simulink model "dandianji"  (R2014b)
settings: Solver=ode45  StartTime=0.0  StopTime=10.0  RelTol=1e-3
undefined symbols (not defined in the file): sigbuilder_block
libraries: simulink x33, fuzblock x16
(part 1 of 2)
settings Model: Creator=Administrator  LastModifiedBy=Administrator

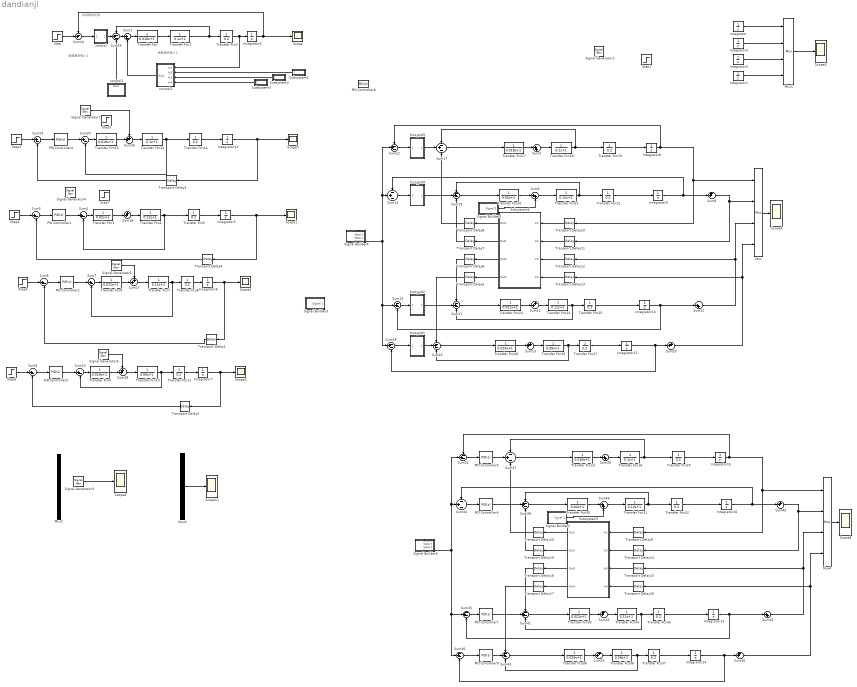
== system dandianji ==
  note: 偏差耦合输入2
  note: 系统原有反馈
  note: 偏差耦合输入1
  Integrator{,1..16} (17 alike) : Integrator
  Mux{,1..4} (5 alike) : Mux
  PID Controller1 : simulink/Continuous/PID Controller  Controller=PID  TimeDomain=Continuous-time  SampleTime=-1  IntegratorMethod=Forward Euler  FilterMethod=Forward Euler  Form=Parallel  P=4.34348893595362  I=0.409606906541511  D=0.190106280421876  N=113.521570556965  InitialConditionSource=internal  InitialConditionForIntegrator=0  InitialConditionForFilter=0  ExternalReset=none  LimitOutput=off  UpperSaturationLimit=inf  LowerSaturationLimit=-inf  LinearizeAsGain=on  AntiWindupMode=none  Kb=1  TrackingMode=off  Kt=1  PParamMin=[]  PParamMax=[]  IParamMin=[]  IParamMax=[]  DParamMin=[]  DParamMax=[]  NParamMin=[]  NParamMax=[]  KbParamMin=[]  KbParamMax=[]  KtParamMin=[]  KtParamMax=[]  POutMin=[]  POutMax=[]  IOutMin=[]  IOutMax=[]  DOutMin=[]  DOutMax=[]  NOutMin=[]  NOutMax=[]  KbOutMin=[]  KbOutMax=[]  KtOutMin=[]  KtOutMax=[]  IntegratorOutMin=[]  IntegratorOutMax=[]  FilterOutMin=[]  FilterOutMax=[]  SumOutMin=[]  SumOutMax=[]  SumI1OutMin=[]  SumI1OutMax=[]  SumI2OutMin=[]  SumI2OutMax=[]  SumI3OutMin=[]  SumI3OutMax=[]  SumDOutMin=[]  SumDOutMax=[]  SaturationOutMin=[]  SaturationOutMax=[]  IntegratorContinuousStateAttributes=''  IntegratorStateMustResolveToSignalObject=off  IntegratorRTWStateStorageClass=Auto  FilterContinuousStateAttributes=''  FilterStateMustResolveToSignalObject=off  FilterRTWStateStorageClass=Auto  DifferentiatorICPrevScaledInput=0  DifferentiatorOutMin=[]  DifferentiatorOutMax=[]  UseFilter=on
  PID Controller2 : simulink/Continuous/PID Controller  Controller=PID  TimeDomain=Continuous-time  SampleTime=-1  IntegratorMethod=Forward Euler  FilterMethod=Forward Euler  Form=Parallel  P=4.3714761921553  I=0.418612157121434  D=0.176716531069936  N=115.244644738995  InitialConditionSource=internal  InitialConditionForIntegrator=0  InitialConditionForFilter=0  ExternalReset=none  LimitOutput=off  UpperSaturationLimit=inf  LowerSaturationLimit=-inf  LinearizeAsGain=on  AntiWindupMode=none  Kb=1  TrackingMode=off  Kt=1  PParamMin=[]  PParamMax=[]  IParamMin=[]  IParamMax=[]  DParamMin=[]  DParamMax=[]  NParamMin=[]  NParamMax=[]  KbParamMin=[]  KbParamMax=[]  KtParamMin=[]  KtParamMax=[]  POutMin=[]  POutMax=[]  IOutMin=[]  IOutMax=[]  DOutMin=[]  DOutMax=[]  NOutMin=[]  NOutMax=[]  KbOutMin=[]  KbOutMax=[]  KtOutMin=[]  KtOutMax=[]  IntegratorOutMin=[]  IntegratorOutMax=[]  FilterOutMin=[]  FilterOutMax=[]  SumOutMin=[]  SumOutMax=[]  SumI1OutMin=[]  SumI1OutMax=[]  SumI2OutMin=[]  SumI2OutMax=[]  SumI3OutMin=[]  SumI3OutMax=[]  SumDOutMin=[]  SumDOutMax=[]  SaturationOutMin=[]  SaturationOutMax=[]  IntegratorContinuousStateAttributes=''  IntegratorStateMustResolveToSignalObject=off  IntegratorRTWStateStorageClass=Auto  FilterContinuousStateAttributes=''  FilterStateMustResolveToSignalObject=off  FilterRTWStateStorageClass=Auto  DifferentiatorICPrevScaledInput=0  DifferentiatorOutMin=[]  DifferentiatorOutMax=[]  UseFilter=on
  PID Controller3 : simulink/Continuous/PID Controller  Controller=PID  TimeDomain=Continuous-time  SampleTime=-1  IntegratorMethod=Forward Euler  FilterMethod=Forward Euler  Form=Parallel  P=4.54060551459518  I=0.450019772467081  D=0.137661903224342  N=119.172045893014  InitialConditionSource=internal  InitialConditionForIntegrator=0  InitialConditionForFilter=0  ExternalReset=none  LimitOutput=off  UpperSaturationLimit=inf  LowerSaturationLimit=-inf  LinearizeAsGain=on  AntiWindupMode=none  Kb=1  TrackingMode=off  Kt=1  PParamMin=[]  PParamMax=[]  IParamMin=[]  IParamMax=[]  DParamMin=[]  DParamMax=[]  NParamMin=[]  NParamMax=[]  KbParamMin=[]  KbParamMax=[]  KtParamMin=[]  KtParamMax=[]  POutMin=[]  POutMax=[]  IOutMin=[]  IOutMax=[]  DOutMin=[]  DOutMax=[]  NOutMin=[]  NOutMax=[]  KbOutMin=[]  KbOutMax=[]  KtOutMin=[]  KtOutMax=[]  IntegratorOutMin=[]  IntegratorOutMax=[]  FilterOutMin=[]  FilterOutMax=[]  SumOutMin=[]  SumOutMax=[]  SumI1OutMin=[]  SumI1OutMax=[]  SumI2OutMin=[]  SumI2OutMax=[]  SumI3OutMin=[]  SumI3OutMax=[]  SumDOutMin=[]  SumDOutMax=[]  SaturationOutMin=[]  SaturationOutMax=[]  IntegratorContinuousStateAttributes=''  IntegratorStateMustResolveToSignalObject=off  IntegratorRTWStateStorageClass=Auto  FilterContinuousStateAttributes=''  FilterStateMustResolveToSignalObject=off  FilterRTWStateStorageClass=Auto  DifferentiatorICPrevScaledInput=0  DifferentiatorOutMin=[]  DifferentiatorOutMax=[]  UseFilter=on
  PID Controller4 : simulink/Continuous/PID Controller  Controller=PID  TimeDomain=Continuous-time  SampleTime=-1  IntegratorMethod=Forward Euler  FilterMethod=Forward Euler  Form=Parallel  P=4.45385591758043  I=0.428539114293849  D=0.147050814476134  N=115.714109449814  InitialConditionSource=internal  InitialConditionForIntegrator=0  InitialConditionForFilter=0  ExternalReset=none  LimitOutput=off  UpperSaturationLimit=inf  LowerSaturationLimit=-inf  LinearizeAsGain=on  AntiWindupMode=none  Kb=1  TrackingMode=off  Kt=1  PParamMin=[]  PParamMax=[]  IParamMin=[]  IParamMax=[]  DParamMin=[]  DParamMax=[]  NParamMin=[]  NParamMax=[]  KbParamMin=[]  KbParamMax=[]  KtParamMin=[]  KtParamMax=[]  POutMin=[]  POutMax=[]  IOutMin=[]  IOutMax=[]  DOutMin=[]  DOutMax=[]  NOutMin=[]  NOutMax=[]  KbOutMin=[]  KbOutMax=[]  KtOutMin=[]  KtOutMax=[]  IntegratorOutMin=[]  IntegratorOutMax=[]  FilterOutMin=[]  FilterOutMax=[]  SumOutMin=[]  SumOutMax=[]  SumI1OutMin=[]  SumI1OutMax=[]  SumI2OutMin=[]  SumI2OutMax=[]  SumI3OutMin=[]  SumI3OutMax=[]  SumDOutMin=[]  SumDOutMax=[]  SaturationOutMin=[]  SaturationOutMax=[]  IntegratorContinuousStateAttributes=''  IntegratorStateMustResolveToSignalObject=off  IntegratorRTWStateStorageClass=Auto  FilterContinuousStateAttributes=''  FilterStateMustResolveToSignalObject=off  FilterRTWStateStorageClass=Auto  DifferentiatorICPrevScaledInput=0  DifferentiatorOutMin=[]  DifferentiatorOutMax=[]  UseFilter=on
  PID Controller5 : simulink/Continuous/PID Controller  Controller=PID  TimeDomain=Continuous-time  SampleTime=-1  IntegratorMethod=Forward Euler  FilterMethod=Forward Euler  Form=Parallel  P=4.45385591758043  I=0.428539114293849  D=0.147050814476134  N=115.714109449814  InitialConditionSource=internal  InitialConditionForIntegrator=0  InitialConditionForFilter=0  ExternalReset=none  LimitOutput=off  UpperSaturationLimit=inf  LowerSaturationLimit=-inf  LinearizeAsGain=on  AntiWindupMode=none  Kb=1  TrackingMode=off  Kt=1  PParamMin=[]  PParamMax=[]  IParamMin=[]  IParamMax=[]  DParamMin=[]  DParamMax=[]  NParamMin=[]  NParamMax=[]  KbParamMin=[]  KbParamMax=[]  KtParamMin=[]  KtParamMax=[]  POutMin=[]  POutMax=[]  IOutMin=[]  IOutMax=[]  DOutMin=[]  DOutMax=[]  NOutMin=[]  NOutMax=[]  KbOutMin=[]  KbOutMax=[]  KtOutMin=[]  KtOutMax=[]  IntegratorOutMin=[]  IntegratorOutMax=[]  FilterOutMin=[]  FilterOutMax=[]  SumOutMin=[]  SumOutMax=[]  SumI1OutMin=[]  SumI1OutMax=[]  SumI2OutMin=[]  SumI2OutMax=[]  SumI3OutMin=[]  SumI3OutMax=[]  SumDOutMin=[]  SumDOutMax=[]  SaturationOutMin=[]  SaturationOutMax=[]  IntegratorContinuousStateAttributes=''  IntegratorStateMustResolveToSignalObject=off  IntegratorRTWStateStorageClass=Auto  FilterContinuousStateAttributes=''  FilterStateMustResolveToSignalObject=off  FilterRTWStateStorageClass=Auto  DifferentiatorICPrevScaledInput=0  DifferentiatorOutMin=[]  DifferentiatorOutMax=[]  UseFilter=on
  PID Controller6 : simulink/Continuous/PID Controller  Controller=PID  TimeDomain=Continuous-time  SampleTime=-1  IntegratorMethod=Forward Euler  FilterMethod=Forward Euler  Form=Parallel  P=4.34348893595362  I=0.409606906541511  D=0.190106280421876  N=113.521570556965  InitialConditionSource=internal  InitialConditionForIntegrator=0  InitialConditionForFilter=0  ExternalReset=none  LimitOutput=off  UpperSaturationLimit=inf  LowerSaturationLimit=-inf  LinearizeAsGain=on  AntiWindupMode=none  Kb=1  TrackingMode=off  Kt=1  PParamMin=[]  PParamMax=[]  IParamMin=[]  IParamMax=[]  DParamMin=[]  DParamMax=[]  NParamMin=[]  NParamMax=[]  KbParamMin=[]  KbParamMax=[]  KtParamMin=[]  KtParamMax=[]  POutMin=[]  POutMax=[]  IOutMin=[]  IOutMax=[]  DOutMin=[]  DOutMax=[]  NOutMin=[]  NOutMax=[]  KbOutMin=[]  KbOutMax=[]  KtOutMin=[]  KtOutMax=[]  IntegratorOutMin=[]  IntegratorOutMax=[]  FilterOutMin=[]  FilterOutMax=[]  SumOutMin=[]  SumOutMax=[]  SumI1OutMin=[]  SumI1OutMax=[]  SumI2OutMin=[]  SumI2OutMax=[]  SumI3OutMin=[]  SumI3OutMax=[]  SumDOutMin=[]  SumDOutMax=[]  SaturationOutMin=[]  SaturationOutMax=[]  IntegratorContinuousStateAttributes=''  IntegratorStateMustResolveToSignalObject=off  IntegratorRTWStateStorageClass=Auto  FilterContinuousStateAttributes=''  FilterStateMustResolveToSignalObject=off  FilterRTWStateStorageClass=Auto  DifferentiatorICPrevScaledInput=0  DifferentiatorOutMin=[]  DifferentiatorOutMax=[]  UseFilter=on
  PID Controller7 : simulink/Continuous/PID Controller  Controller=PID  TimeDomain=Continuous-time  SampleTime=-1  IntegratorMethod=Forward Euler  FilterMethod=Forward Euler  Form=Parallel  P=4.3714761921553  I=0.418612157121434  D=0.176716531069936  N=115.244644738995  InitialConditionSource=internal  InitialConditionForIntegrator=0  InitialConditionForFilter=0  ExternalReset=none  LimitOutput=off  UpperSaturationLimit=inf  LowerSaturationLimit=-inf  LinearizeAsGain=on  AntiWindupMode=none  Kb=1  TrackingMode=off  Kt=1  PParamMin=[]  PParamMax=[]  IParamMin=[]  IParamMax=[]  DParamMin=[]  DParamMax=[]  NParamMin=[]  NParamMax=[]  KbParamMin=[]  KbParamMax=[]  KtParamMin=[]  KtParamMax=[]  POutMin=[]  POutMax=[]  IOutMin=[]  IOutMax=[]  DOutMin=[]  DOutMax=[]  NOutMin=[]  NOutMax=[]  KbOutMin=[]  KbOutMax=[]  KtOutMin=[]  KtOutMax=[]  IntegratorOutMin=[]  IntegratorOutMax=[]  FilterOutMin=[]  FilterOutMax=[]  SumOutMin=[]  SumOutMax=[]  SumI1OutMin=[]  SumI1OutMax=[]  SumI2OutMin=[]  SumI2OutMax=[]  SumI3OutMin=[]  SumI3OutMax=[]  SumDOutMin=[]  SumDOutMax=[]  SaturationOutMin=[]  SaturationOutMax=[]  IntegratorContinuousStateAttributes=''  IntegratorStateMustResolveToSignalObject=off  IntegratorRTWStateStorageClass=Auto  FilterContinuousStateAttributes=''  FilterStateMustResolveToSignalObject=off  FilterRTWStateStorageClass=Auto  DifferentiatorICPrevScaledInput=0  DifferentiatorOutMin=[]  DifferentiatorOutMax=[]  UseFilter=on
  PID Controller8 : simulink/Continuous/PID Controller  Controller=PID  TimeDomain=Continuous-time  SampleTime=-1  IntegratorMethod=Forward Euler  FilterMethod=Forward Euler  Form=Parallel  P=12.9851074749726  I=3.96505413373294  D=0.756963167778154  N=4061.73491108422  InitialConditionSource=internal  InitialConditionForIntegrator=0  InitialConditionForFilter=0  ExternalReset=none  LimitOutput=off  UpperSaturationLimit=inf  LowerSaturationLimit=-inf  LinearizeAsGain=on  AntiWindupMode=none  Kb=1  TrackingMode=off  Kt=1  PParamMin=[]  PParamMax=[]  IParamMin=[]  IParamMax=[]  DParamMin=[]  DParamMax=[]  NParamMin=[]  NParamMax=[]  KbParamMin=[]  KbParamMax=[]  KtParamMin=[]  KtParamMax=[]  POutMin=[]  POutMax=[]  IOutMin=[]  IOutMax=[]  DOutMin=[]  DOutMax=[]  NOutMin=[]  NOutMax=[]  KbOutMin=[]  KbOutMax=[]  KtOutMin=[]  KtOutMax=[]  IntegratorOutMin=[]  IntegratorOutMax=[]  FilterOutMin=[]  FilterOutMax=[]  SumOutMin=[]  SumOutMax=[]  SumI1OutMin=[]  SumI1OutMax=[]  SumI2OutMin=[]  SumI2OutMax=[]  SumI3OutMin=[]  SumI3OutMax=[]  SumDOutMin=[]  SumDOutMax=[]  SaturationOutMin=[]  SaturationOutMax=[]  IntegratorContinuousStateAttributes=''  IntegratorStateMustResolveToSignalObject=off  IntegratorRTWStateStorageClass=Auto  FilterContinuousStateAttributes=''  FilterStateMustResolveToSignalObject=off  FilterRTWStateStorageClass=Auto  DifferentiatorICPrevScaledInput=0  DifferentiatorOutMin=[]  DifferentiatorOutMax=[]  UseFilter=on
  PID Controller9 : simulink/Continuous/PID Controller  Controller=PID  TimeDomain=Continuous-time  SampleTime=-1  IntegratorMethod=Forward Euler  FilterMethod=Forward Euler  Form=Parallel  P=4.54060551459518  I=0.450019772467081  D=0.137661903224342  N=119.172045893014  InitialConditionSource=internal  InitialConditionForIntegrator=0  InitialConditionForFilter=0  ExternalReset=none  LimitOutput=off  UpperSaturationLimit=inf  LowerSaturationLimit=-inf  LinearizeAsGain=on  AntiWindupMode=none  Kb=1  TrackingMode=off  Kt=1  PParamMin=[]  PParamMax=[]  IParamMin=[]  IParamMax=[]  DParamMin=[]  DParamMax=[]  NParamMin=[]  NParamMax=[]  KbParamMin=[]  KbParamMax=[]  KtParamMin=[]  KtParamMax=[]  POutMin=[]  POutMax=[]  IOutMin=[]  IOutMax=[]  DOutMin=[]  DOutMax=[]  NOutMin=[]  NOutMax=[]  KbOutMin=[]  KbOutMax=[]  KtOutMin=[]  KtOutMax=[]  IntegratorOutMin=[]  IntegratorOutMax=[]  FilterOutMin=[]  FilterOutMax=[]  SumOutMin=[]  SumOutMax=[]  SumI1OutMin=[]  SumI1OutMax=[]  SumI2OutMin=[]  SumI2OutMax=[]  SumI3OutMin=[]  SumI3OutMax=[]  SumDOutMin=[]  SumDOutMax=[]  SaturationOutMin=[]  SaturationOutMax=[]  IntegratorContinuousStateAttributes=''  IntegratorStateMustResolveToSignalObject=off  IntegratorRTWStateStorageClass=Auto  FilterContinuousStateAttributes=''  FilterStateMustResolveToSignalObject=off  FilterRTWStateStorageClass=Auto  DifferentiatorICPrevScaledInput=0  DifferentiatorOutMin=[]  DifferentiatorOutMax=[]  UseFilter=on
  Scope{,1..8,11} (10 alike) : Scope
      Scope settings: SaveName=dianji1
      Scope1 settings: SaveName=dianji2
      Scope11 settings: YMin=260  YMax=460  SaveName=wuraodongweizhi5
      Scope2 settings: SaveName=dianji3
      Scope3 settings: SaveName=dianji4
      Scope4 settings: YMin=4.94  YMax=5.02  SaveName=perfect
      Scope5 settings: YMin=260  YMax=460  SaveName=wuraodongweizhi
      Scope6 settings: YMin=-500  YMax=2000  SaveName=wuraodongweizhi1
      Scope7 settings: SaveName=dianji
      Scope8 settings: YMin=4.7  YMax=5.4  SaveName=perfect1
  Signal Generator{1,4..6} (4 alike) : SignalGenerator  WaveForm=random  Amplitude=10  Frequency=2
  Signal Generator2 : SignalGenerator  WaveForm=random  Frequency=2
  Signal Generator3 : SignalGenerator  WaveForm=random  Frequency=2
  Signal Builder1 : Subsystem  Tag=STV Subsys  LoadFcn=sigbuilder_block('load');  StartFcn=sigbuilder_block('start');  StopFcn=sigbuilder_block('stop');  ClipboardFcn=sigbuilder_block('clipboard');  mask(Sigbuilder block){}
      mask help: Simulink:masks:SigbuilderBlock_MD
      mask init:
      | if ~strcmp(get_param(bdroot(gcbh),'SimulationStatus'),'stopped') tuvar = sigbuilder_block('maskInit'); end
      settings: CopyFcn=sigbuilder_block('copy');  DeleteFcn=sigbuilder_block('delete');  ModelCloseFcn=sigbuilder_block('modelClose');  PreSaveFcn=sigbuilder_block('preSave');  PauseFcn=sigbuilder_block('pause');  ContinueFcn=sigbuilder_block('continue');  NameChangeFcn=sigbuilder_block('namechange');  OpenFcn=sigbuilder_block('open',[437.6 199.2 550.4 400 ]);  CloseFcn=sigbuilder_block('close');
      mask Display: plot(0, 0, 100, 100,[2, 2, 32, 32, 2], [68, 8, 8, 68, 68],[32, 2], [38, 38], [32, 19, 2],[53, 60, 44], [32, 17, 17, 2],[16, 16, 31, 31]);txt = getActiveGroup(gcbh);text(2, 100, txt,'verticalAlignment', 'top');
  Signal Builder2 : Subsystem  Tag=STV Subsys  LoadFcn=sigbuilder_block('load');  StartFcn=sigbuilder_block('start');  StopFcn=sigbuilder_block('stop');  ClipboardFcn=sigbuilder_block('clipboard');  mask(Sigbuilder block){}
      mask help: Simulink:masks:SigbuilderBlock_MD
      mask init:
      | if ~strcmp(get_param(bdroot(gcbh),'SimulationStatus'),'stopped') tuvar = sigbuilder_block('maskInit'); end
      settings: CopyFcn=sigbuilder_block('copy');  DeleteFcn=sigbuilder_block('delete');  ModelCloseFcn=sigbuilder_block('modelClose');  PreSaveFcn=sigbuilder_block('preSave');  PauseFcn=sigbuilder_block('pause');  ContinueFcn=sigbuilder_block('continue');  NameChangeFcn=sigbuilder_block('namechange');  OpenFcn=sigbuilder_block('open',[437.6 199.2 550.4 400 ]);  CloseFcn=sigbuilder_block('close');
      mask Display: plot(0, 0, 100, 100,[2, 2, 32, 32, 2], [68, 8, 8, 68, 68],[32, 2], [38, 38], [32, 19, 2],[53, 60, 44], [32, 17, 17, 2],[16, 16, 31, 31]);txt = getActiveGroup(gcbh);text(2, 100, txt,'verticalAlignment', 'top');
  Signal Builder3 : Subsystem  Tag=STV Subsys  LoadFcn=sigbuilder_block('load');  StartFcn=sigbuilder_block('start');  StopFcn=sigbuilder_block('stop');  ClipboardFcn=sigbuilder_block('clipboard');  mask(Sigbuilder block){}
      mask help: Simulink:masks:SigbuilderBlock_MD
      mask init:
      | if ~strcmp(get_param(bdroot(gcbh),'SimulationStatus'),'stopped') tuvar = sigbuilder_block('maskInit'); end
      settings: CopyFcn=sigbuilder_block('copy');  DeleteFcn=sigbuilder_block('delete');  ModelCloseFcn=sigbuilder_block('modelClose');  PreSaveFcn=sigbuilder_block('preSave');  PauseFcn=sigbuilder_block('pause');  ContinueFcn=sigbuilder_block('continue');  NameChangeFcn=sigbuilder_block('namechange');  OpenFcn=sigbuilder_block('open',[437.6 199.2 550.4 400 ]);  CloseFcn=sigbuilder_block('close');
      mask Display: plot(0, 0, 100, 100,[2, 2, 32, 32, 2], [68, 8, 8, 68, 68],[32, 2], [38, 38], [32, 19, 2],[53, 60, 44], [32, 17, 17, 2],[16, 16, 31, 31]);txt = getActiveGroup(gcbh);text(2, 100, txt,'verticalAlignment', 'top');
  Signal Builder4 : Subsystem  Tag=STV Subsys  LoadFcn=sigbuilder_block('load');  StartFcn=sigbuilder_block('start');  StopFcn=sigbuilder_block('stop');  ClipboardFcn=sigbuilder_block('clipboard');  mask(Sigbuilder block){}
      mask help: Simulink:masks:SigbuilderBlock_MD
      mask init:
      | if ~strcmp(get_param(bdroot(gcbh),'SimulationStatus'),'stopped') tuvar = sigbuilder_block('maskInit'); end
      settings: CopyFcn=sigbuilder_block('copy');  DeleteFcn=sigbuilder_block('delete');  ModelCloseFcn=sigbuilder_block('modelClose');  PreSaveFcn=sigbuilder_block('preSave');  PauseFcn=sigbuilder_block('pause');  ContinueFcn=sigbuilder_block('continue');  NameChangeFcn=sigbuilder_block('namechange');  OpenFcn=sigbuilder_block('open',[437.6 199.2 550.4 400 ]);  CloseFcn=sigbuilder_block('close');
      mask Display: plot(0, 0, 100, 100,[2, 2, 32, 32, 2], [68, 8, 8, 68, 68],[32, 2], [38, 38], [32, 19, 2],[53, 60, 44], [32, 17, 17, 2],[16, 16, 31, 31]);txt = getActiveGroup(gcbh);text(2, 100, txt,'verticalAlignment', 'top');
  Signal Builder5 : Subsystem  Tag=STV Subsys  LoadFcn=sigbuilder_block('load');  StartFcn=sigbuilder_block('start');  StopFcn=sigbuilder_block('stop');  ClipboardFcn=sigbuilder_block('clipboard');  mask(Sigbuilder block){}
      mask help: Simulink:masks:SigbuilderBlock_MD
      mask init:
      | if ~strcmp(get_param(bdroot(gcbh),'SimulationStatus'),'stopped') tuvar = sigbuilder_block('maskInit'); end
      settings: CopyFcn=sigbuilder_block('copy');  DeleteFcn=sigbuilder_block('delete');  ModelCloseFcn=sigbuilder_block('modelClose');  PreSaveFcn=sigbuilder_block('preSave');  PauseFcn=sigbuilder_block('pause');  ContinueFcn=sigbuilder_block('continue');  NameChangeFcn=sigbuilder_block('namechange');  OpenFcn=sigbuilder_block('open',[437.6 199.2 550.4 400 ]);  CloseFcn=sigbuilder_block('close');
      mask Display: plot(0, 0, 100, 100,[2, 2, 32, 32, 2], [68, 8, 8, 68, 68],[32, 2], [38, 38], [32, 19, 2],[53, 60, 44], [32, 17, 17, 2],[16, 16, 31, 31]);txt = getActiveGroup(gcbh);text(2, 100, txt,'verticalAlignment', 'top');
  Step : Step  SampleTime=0
  Step1 : Step  Time=3  SampleTime=0
  Step2 : Step  After=50  SampleTime=0
  Step3 : Step  After=50  SampleTime=0
  Step4 : Step  SampleTime=0
  Step5 : Step  Time=5  After=-1  SampleTime=0
  Step6 : Step  SampleTime=0
  Step7 : Step  Time=5  After=-1  SampleTime=0
  Subsystem1 : Subsystem
  Subsystem2 : Subsystem
  Subsystem3 : Subsystem
  Subsystem4 : Subsystem
  Subsystem5 : Subsystem
  Sum{1,3..4,6..7,9..10,29..30} (9 alike) : Sum  Inputs=|+-
  Sum{8,11,13,18,20,26..28,31,33,40,45} (12 alike) : Sum  Inputs=++|
  Sum{12,14..17,19,21,23,25,32,34..38,41,43} (17 alike) : Sum  Inputs=-+-
  Sum{2,5,22,39,42,44} (6 alike) : Sum  Inputs=|++
  Sum24 : Sum  Inputs=-+|
  Transfer Fcn{,13,15,17} (4 alike) : TransferFcn  Denominator=[0.018 1]
  Transfer Fcn{1,12,16,18} (4 alike) : TransferFcn  Denominator=[0.1 1]
  Transfer Fcn10 : TransferFcn  Denominator=[0.09 1]
  Transfer Fcn{2,5,8,11,14,19,22,25,27,29,32,35,37} (13 alike) : TransferFcn  Denominator=[0.2]
  Transfer Fcn20 : TransferFcn  Denominator=[0.02 1]
  Transfer Fcn21 : TransferFcn  Denominator=[0.12 1]
  Transfer Fcn23 : TransferFcn  Denominator=[0.021 1]
  Transfer Fcn24 : TransferFcn  Denominator=[0.11 1]
  Transfer Fcn26 : TransferFcn  Denominator=[0.09 1]
  Transfer Fcn28 : TransferFcn  Denominator=[0.019 1]
  Transfer Fcn3 : TransferFcn  Denominator=[0.02 1]
  Transfer Fcn30 : TransferFcn  Denominator=[0.02 1]
  Transfer Fcn31 : TransferFcn  Denominator=[0.12 1]
  Transfer Fcn33 : TransferFcn  Denominator=[0.021 1]
  Transfer Fcn34 : TransferFcn  Denominator=[0.11 1]
  Transfer Fcn36 : TransferFcn  Denominator=[0.09 1]
  Transfer Fcn38 : TransferFcn  Denominator=[0.019 1]
  Transfer Fcn4 : TransferFcn  Denominator=[0.12 1]
  Transfer Fcn6 : TransferFcn  Denominator=[0.021 1]
  Transfer Fcn7 : TransferFcn  Denominator=[0.11 1]
  Transfer Fcn9 : TransferFcn  Denominator=[0.019 1]
  Transport Delay{1..4} (4 alike) : TransportDelay  DelayTime=0.02
  Transport Delay{5..16} (12 alike) : TransportDelay  DelayTime=0.001
  Transport Delay17 : TransportDelay  DelayTime=0.003
  Transport Delay18 : TransportDelay  DelayTime=0.005
  Transport Delay19 : TransportDelay  DelayTime=0.003
  Transport Delay20 : TransportDelay  DelayTime=0.003
  control : Subsystem
  control1 : Subsystem
  control2 : Subsystem
  fuzzypid1 : Subsystem
  fuzzypid2 : Subsystem
  fuzzypid3 : Subsystem
  fuzzypid4 : Subsystem
  wires:
  Transfer Fcn1/1 -> Transfer Fcn2/1, Sum25/1
  Transfer Fcn/1 -> Transfer Fcn1/1
  Step2/1 -> Sum3/1
  Sum3/1 -> PID Controller1/1
  Transfer Fcn4/1 -> Sum4/2, Transfer Fcn5/1
  Sum4/1 -> Transfer Fcn3/1
  PID Controller1/1 -> Sum4/1
  Transfer Fcn5/1 -> Integrator5/1
  Step4/1 -> Sum6/1
  Sum6/1 -> PID Controller2/1
  Transfer Fcn7/1 -> Transfer Fcn8/1, Sum7/2
  Sum7/1 -> Transfer Fcn6/1
  PID Controller2/1 -> Sum7/1
  Transfer Fcn8/1 -> Integrator6/1
  Step6/1 -> Sum9/1
  Sum9/1 -> PID Controller3/1
  Transfer Fcn10/1 -> Transfer Fcn11/1, Sum10/2
  Sum10/1 -> Transfer Fcn9/1
  PID Controller3/1 -> Sum10/1
  Transfer Fcn11/1 -> Integrator7/1
  Mux/1 -> Scope4/1
  Mux1/1 -> Scope5/1
  Signal Builder4/4(Signal 1) -> Sum12/2, Sum14/2, Sum15/2, Sum16/2
  Transfer Fcn19/1 -> Integrator8/1
  Transfer Fcn22/1 -> Integrator9/1
  Transfer Fcn25/1 -> Integrator10/1
  Transfer Fcn27/1 -> Integrator11/1
  Transfer Fcn2/1 -> control2/1(In1), Integrator4/1
  Transfer Fcn18/1 -> Transfer Fcn19/1, Sum17/1
  Sum17/1 -> Transfer Fcn17/1
  Transfer Fcn21/1 -> Transfer Fcn22/1, Sum19/1
  Sum19/1 -> Transfer Fcn20/1
  Sum21/1 -> Transfer Fcn23/1
  Transfer Fcn24/1 -> Sum21/3, Transfer Fcn25/1
  Transfer Fcn26/1 -> Sum23/3, Transfer Fcn27/1
  Sum23/1 -> Transfer Fcn28/1
  Integrator/1 -> Mux1/1
  Integrator3/1 -> Mux1/2
  Integrator2/1 -> Mux1/3
  Integrator1/1 -> Mux1/4
  Integrator4/1 -> Sum24/1, Scope/1
  Integrator6/1 -> Scope2/1, Transport Delay1/1
  Integrator7/1 -> Scope3/1, Transport Delay2/1
  Integrator8/1 -> Transport Delay10/1, Mux/1, Sum12/1
  Integrator9/1 -> Sum8/2, Sum14/1
  Integrator10/1 -> Sum22/1, Sum15/3
  Transfer Fcn17/1 -> Sum2/1
  Sum2/1 -> Transfer Fcn18/1
  Transfer Fcn20/1 -> Sum5/1
  Sum5/1 -> Transfer Fcn21/1
  Sum13/1 -> Transfer Fcn26/1
  Transfer Fcn28/1 -> Sum13/2
  Sum8/1 -> Transport Delay11/1, Mux/2
  Sum22/1 -> Transport Delay12/1, Mux/3
  Sum20/1 -> Transport Delay13/1, Mux/4
  Integrator11/1 -> Sum20/2, Sum16/3
  Transfer Fcn3/1 -> Sum18/2
  Sum18/1 -> Transfer Fcn4/1
  Signal Generator3/1 -> Scope6/1
  Subsystem4/4(Out4) -> Transport Delay5/1
  Subsystem4/3(Out3) -> Transport Delay6/1
  Subsystem4/1(Out1) -> Transport Delay8/1
  Mux3/1 -> Scope11/1
  Sum11/1 -> Transfer Fcn24/1
  Transfer Fcn23/1 -> Sum11/2
  Integrator5/1 -> Scope1/1, Transport Delay4/1
  Transport Delay4/1 -> Sum3/2
  Subsystem4/2(Out2) -> Transport Delay7/1
  Transport Delay1/1 -> Sum6/2
  Transport Delay2/1 -> Sum9/2
  Signal Generator5/1 -> Sum27/1
  Transfer Fcn6/1 -> Sum27/2
  Sum27/1 -> Transfer Fcn7/1
  Transfer Fcn9/1 -> Sum28/2
  Sum28/1 -> Transfer Fcn10/1
  Signal Generator6/1 -> Sum28/1
  Transport Delay10/1 -> Subsystem4/1(In1)
  Transport Delay11/1 -> Subsystem4/2(In2)
  Transport Delay12/1 -> Subsystem4/3(In3)
  Transport Delay13/1 -> Subsystem4/4(In4)
  control/1(Out1) -> Sum25/2
  fuzzypid3/1(Out1) -> Sum17/2
  Sum12/1 -> fuzzypid3/1(In1)
  Sum14/1 -> fuzzypid4/1(In1)
  fuzzypid4/1(Out1) -> Sum19/2
  Sum15/1 -> fuzzypid2/1(In1)
  fuzzypid2/1(Out1) -> Sum21/2
  Sum16/1 -> fuzzypid1/1(In1)
  fuzzypid1/1(Out1) -> Sum23/2
  Signal Builder2/1(Signal 2) -> Sum5/2
  Step/1 -> Sum24/2
  Sum24/1 -> control/1(In1)
  Subsystem1/1(Out1) -> control2/2(In2)
  Subsystem2/1(Out1) -> control2/3(In3)
  Subsystem3/1(Out1) -> control2/4(In4)
  Transport Delay8/1 -> Sum17/3
  Transport Delay7/1 -> Sum19/3
  Transport Delay6/1 -> Sum21/1
  Transport Delay5/1 -> Sum23/1
  Sum25/1 -> Sum1/1
  Sum1/1 -> Transfer Fcn/1
  control1/1(Out1) -> Sum25/3
  control2/1(Out1) -> Sum1/2
  Step3/1 -> Sum29/1
  Sum29/1 -> PID Controller4/1
  Transfer Fcn12/1 -> Sum30/2, Transfer Fcn14/1
  Sum30/1 -> Transfer Fcn15/1
  PID Controller4/1 -> Sum30/1
  Transfer Fcn14/1 -> Integrator12/1
  Sum26/1 -> Transfer Fcn12/1
  Integrator12/1 -> Transport Delay3/1, Scope7/1
  Signal Generator1/1 -> Sum26/1
  Transport Delay3/1 -> Sum29/2
  Transfer Fcn15/1 -> Sum26/2
  Mux4/1 -> Scope8/1
  Signal Builder5/4(Signal 1) -> Sum32/2, Sum34/2, Sum35/2, Sum36/2
  Transfer Fcn29/1 -> Integrator15/1
  Transfer Fcn32/1 -> Integrator16/1
  Transfer Fcn35/1 -> Integrator13/1
  Transfer Fcn37/1 -> Integrator14/1
  Transfer Fcn16/1 -> Transfer Fcn29/1, Sum37/1
  Sum37/1 -> Transfer Fcn13/1
  Transfer Fcn31/1 -> Transfer Fcn32/1, Sum38/1
  Sum38/1 -> Transfer Fcn30/1
  Sum41/1 -> Transfer Fcn33/1
  Transfer Fcn34/1 -> Sum41/3, Transfer Fcn35/1
  Transfer Fcn36/1 -> Sum43/3, Transfer Fcn37/1
  Sum43/1 -> Transfer Fcn38/1
  Integrator15/1 -> Transport Delay9/1, Mux4/1, Sum32/1
  Integrator16/1 -> Sum45/2, Sum34/1
  Integrator13/1 -> Sum42/1, Sum35/3
  Transfer Fcn13/1 -> Sum39/1
  Sum39/1 -> Transfer Fcn16/1
  Transfer Fcn30/1 -> Sum44/1
  Sum44/1 -> Transfer Fcn31/1
  Sum33/1 -> Transfer Fcn36/1
  Transfer Fcn38/1 -> Sum33/2
  Sum45/1 -> Transport Delay14/1, Mux4/2
  Sum42/1 -> Transport Delay15/1, Mux4/3
  Sum40/1 -> Transport Delay16/1, Mux4/4
  Integrator14/1 -> Sum40/2, Sum36/3
  Subsystem5/4(Out4) -> Transport Delay17/1
  Subsystem5/3(Out3) -> Transport Delay18/1
  Subsystem5/1(Out1) -> Transport Delay20/1
  Sum31/1 -> Transfer Fcn34/1
  Transfer Fcn33/1 -> Sum31/2
  Subsystem5/2(Out2) -> Transport Delay19/1
  Transport Delay9/1 -> Subsystem5/1(In1)
  Transport Delay14/1 -> Subsystem5/2(In2)
  Transport Delay15/1 -> Subsystem5/3(In3)
  Transport Delay16/1 -> Subsystem5/4(In4)
  PID Controller5/1 -> Sum37/2
  Sum32/1 -> PID Controller5/1
  Sum34/1 -> PID Controller6/1
  PID Controller6/1 -> Sum38/2
  Sum35/1 -> PID Controller7/1
  PID Controller7/1 -> Sum41/2
  Sum36/1 -> PID Controller9/1
  PID Controller9/1 -> Sum43/2
  Signal Builder1/1(Signal 2) -> Sum44/2
  Transport Delay20/1 -> Sum37/3
  Transport Delay19/1 -> Sum38/3
  Transport Delay18/1 -> Sum41/1
  Transport Delay17/1 -> Sum43/1

== system dandianji/Signal Builder1 ==
  Demux : Demux  Tag=STV Demux  Outputs=1
  FromWs : FromWorkspace  Tag=STV FromWs  VariableName=tuvar  SampleTime=0
      SigBuilderData=|
      | common.afterFinalStr = 'Extrapolate'
      | common.sampleTime = 0
      | dataSet.timeRange = [0 30]
      | dataSet.name = 'Group 1'
      | sbobj.Groups.Name = 'Group 1'
      | sbobj.Groups.Signals.Name = 'Signal 2'
      | sbobj.Groups.Signals.XData = [0 3.6 3.6 5 5 30]
      | sbobj.Groups.Signals.YData = [0 0 8 8 0 0]
      | sbobj.Groups.TimeRange = [0 30]
  Signal 2 : Outport  Tag=STV Outport
  wires:
  FromWs/1 -> Demux/1
  Demux/1 -> Signal 2/1

== system dandianji/Signal Builder2 ==
  Demux : Demux  Tag=STV Demux  Outputs=1
  FromWs : FromWorkspace  Tag=STV FromWs  VariableName=tuvar  SampleTime=0
      SigBuilderData=|
      | common.afterFinalStr = 'Extrapolate'
      | common.sampleTime = 0
      | dataSet.timeRange = [0 30]
      | dataSet.name = 'Group 1'
      | sbobj.Groups.Name = 'Group 1'
      | sbobj.Groups.Signals.Name = 'Signal 2'
      | sbobj.Groups.Signals.XData = [0 3.6 3.6 5 5 30]
      | sbobj.Groups.Signals.YData = [0 0 8 8 0 0]
      | sbobj.Groups.TimeRange = [0 30]
  Signal 2 : Outport  Tag=STV Outport
  wires:
  FromWs/1 -> Demux/1
  Demux/1 -> Signal 2/1

== system dandianji/Signal Builder3 ==
  Demux : Demux  Tag=STV Demux  Outputs=1
  FromWs : FromWorkspace  Tag=STV FromWs  VariableName=tuvar  SampleTime=0
      SigBuilderData=|
      | common.afterFinalStr = 'Extrapolate'
      | common.sampleTime = 0
      | dataSet.timeRange = [0 10]
      | dataSet.name = 'Group 1'
      | sbobj.Groups.Name = 'Group 1'
      | sbobj.Groups.Signals.Name = 'Signal 1'
      | sbobj.Groups.Signals.XData = [0 7 7 8 8 10]
      | sbobj.Groups.Signals.YData = [0 0 8 8 0 0]
  Signal 1 : Outport  Tag=STV Outport
  wires:
  Demux/1 -> Signal 1/1
  FromWs/1 -> Demux/1

== system dandianji/Signal Builder4 ==
  Demux : Demux  Tag=STV Demux
  FromWs : FromWorkspace  Tag=STV FromWs  VariableName=tuvar  SampleTime=0
      SigBuilderData=|
      | common.afterFinalStr = 'Extrapolate'
      | common.sampleTime = 0
      | dataSet.timeRange = [0 10]
      | dataSet.name = 'Group 1'
      | sbobj.Groups.Name = 'Group 1'
      | sbobj.Groups.Signals(1).Name = 'Signal 2'
      | sbobj.Groups.Signals(1).XData = [0 1.25 1.25 2.5 2.5 3.75 3.75 5 5 6.25 6.25 7.5 7.5 8.75 8.75 10]
      | sbobj.Groups.Signals(1).YData = [30 30 -30 -30 30 30 -30 -30 30 30 -30 -30 30 30 -30 -30]
      | sbobj.Groups.Signals(2).Name = 'Signal 3'
      | sbobj.Groups.Signals(2).XData = [0 5 5 10]
      | sbobj.Groups.Signals(2).YData = [-30 30 -30 -30]
      | sbobj.Groups.Signals(3).Name = 'Signal 4'
      | sbobj.Groups.Signals(3).XData = [0 0.3125 0.625 0.9375 1.25 1.5625 1.875 2.1875 2.5 2.8125 3.125 3.4375 3.75 4.0625 4.375 4.6875 5 5.3125 5.625 5.9375 6.25 6.5625 6.875 7.1875 7.5 7.8125 8.125 8.4375 8.75 9.0625 9.375 9.6875 10]
      | sbobj.Groups.Signals(3).YData = [0 21.2132034356 30 21.2132034356 3.67394039744e-15 -21.2132034356 -30 -21.2132034356 0 21.2132034356 30 21.2132034356 3.67394039744e-15 -21.2132034356 -30 -21.2132034356 0 21.2132034356 30 21.2132034356 3.67394039744e-15 -21.2132034356 -30 -21.2132034356 0 21.2132034356 30 21.2132034356 3.67394039744e-15 -21.2132034356 -30 -21.2132034356 -21.2132034356]
      | sbobj.Groups.Signals(4).Name = 'Signal 1'
      | sbobj.Groups.Signals(4).XData = [0 1 1 10]
      | sbobj.Groups.Signals(4).YData = [0 0 5 5]
  Signal 2 : Outport  Tag=STV Outport
  Signal 3 : Outport  Tag=STV Outport  Port=2
  Signal 4 : Outport  Tag=STV Outport  Port=3
  Signal 1 : Outport  Tag=STV Outport  Port=4
  wires:
  FromWs/1 -> Demux/1
  Demux/1 -> Signal 2/1
  Demux/2 -> Signal 3/1
  Demux/3 -> Signal 4/1
  Demux/4 -> Signal 1/1

== system dandianji/Signal Builder5 ==
  Demux : Demux  Tag=STV Demux
  FromWs : FromWorkspace  Tag=STV FromWs  VariableName=tuvar  SampleTime=0
      SigBuilderData=|
      | common.afterFinalStr = 'Extrapolate'
      | common.sampleTime = 0
      | dataSet.timeRange = [0 10]
      | dataSet.name = 'Group 1'
      | sbobj.Groups.Name = 'Group 1'
      | sbobj.Groups.Signals(1).Name = 'Signal 2'
      | sbobj.Groups.Signals(1).XData = [0 1.25 1.25 2.5 2.5 3.75 3.75 5 5 6.25 6.25 7.5 7.5 8.75 8.75 10]
      | sbobj.Groups.Signals(1).YData = [30 30 -30 -30 30 30 -30 -30 30 30 -30 -30 30 30 -30 -30]
      | sbobj.Groups.Signals(2).Name = 'Signal 3'
      | sbobj.Groups.Signals(2).XData = [0 5 5 10]
      | sbobj.Groups.Signals(2).YData = [-30 30 -30 -30]
      | sbobj.Groups.Signals(3).Name = 'Signal 4'
      | sbobj.Groups.Signals(3).XData = [0 0.3125 0.625 0.9375 1.25 1.5625 1.875 2.1875 2.5 2.8125 3.125 3.4375 3.75 4.0625 4.375 4.6875 5 5.3125 5.625 5.9375 6.25 6.5625 6.875 7.1875 7.5 7.8125 8.125 8.4375 8.75 9.0625 9.375 9.6875 10]
      | sbobj.Groups.Signals(3).YData = [0 21.2132034356 30 21.2132034356 3.67394039744e-15 -21.2132034356 -30 -21.2132034356 0 21.2132034356 30 21.2132034356 3.67394039744e-15 -21.2132034356 -30 -21.2132034356 0 21.2132034356 30 21.2132034356 3.67394039744e-15 -21.2132034356 -30 -21.2132034356 0 21.2132034356 30 21.2132034356 3.67394039744e-15 -21.2132034356 -30 -21.2132034356 -21.2132034356]
      | sbobj.Groups.Signals(4).Name = 'Signal 1'
      | sbobj.Groups.Signals(4).XData = [0 1 1 10]
      | sbobj.Groups.Signals(4).YData = [0 0 5 5]
  Signal 2 : Outport  Tag=STV Outport
  Signal 3 : Outport  Tag=STV Outport  Port=2
  Signal 4 : Outport  Tag=STV Outport  Port=3
  Signal 1 : Outport  Tag=STV Outport  Port=4
  wires:
  FromWs/1 -> Demux/1
  Demux/1 -> Signal 2/1
  Demux/2 -> Signal 3/1
  Demux/3 -> Signal 4/1
  Demux/4 -> Signal 1/1

== system dandianji/Subsystem1 ==
  Out1 : Outport

== system dandianji/Subsystem2 ==
  Out1 : Outport

== system dandianji/Subsystem3 ==
  Out1 : Outport

== system dandianji/Subsystem4 ==
  In1 : Inport
  In2 : Inport  Port=2
  In3 : Inport  Port=3
  In4 : Inport  Port=4
  Subsystem4 : Subsystem
  Subsystem5 : Subsystem
  Subsystem6 : Subsystem
  Subsystem7 : Subsystem
  Out1 : Outport
  Out2 : Outport  Port=2
  Out3 : Outport  Port=3
  Out4 : Outport  Port=4
  wires:
  In1/1 -> Subsystem4/1(In1), Subsystem5/2(In1), Subsystem7/2(In1), Subsystem6/2(In1)
  In2/1 -> Subsystem4/2(In2), Subsystem5/1(In2), Subsystem7/3(In2), Subsystem6/3(In2)
  In3/1 -> Subsystem4/3(In3), Subsystem5/3(In3), Subsystem7/4(In3), Subsystem6/1(In3)
  In4/1 -> Subsystem4/4(In4), Subsystem5/4(In4), Subsystem7/1(In4), Subsystem6/4(In4)
  Subsystem4/1(Out1) -> Out1/1
  Subsystem5/1(Out1) -> Out2/1
  Subsystem6/1(Out1) -> Out3/1
  Subsystem7/1(Out1) -> Out4/1

== system dandianji/Subsystem5 ==
  In1 : Inport
  In2 : Inport  Port=2
  In3 : Inport  Port=3
  In4 : Inport  Port=4
  Subsystem4 : Subsystem
  Subsystem5 : Subsystem
  Subsystem6 : Subsystem
  Subsystem7 : Subsystem
  Out1 : Outport
  Out2 : Outport  Port=2
  Out3 : Outport  Port=3
  Out4 : Outport  Port=4
  wires:
  In1/1 -> Subsystem4/1(In1), Subsystem5/2(In1), Subsystem7/2(In1), Subsystem6/2(In1)
  In2/1 -> Subsystem4/2(In2), Subsystem5/1(In2), Subsystem7/3(In2), Subsystem6/3(In2)
  In3/1 -> Subsystem4/3(In3), Subsystem5/3(In3), Subsystem7/4(In3), Subsystem6/1(In3)
  In4/1 -> Subsystem4/4(In4), Subsystem5/4(In4), Subsystem7/1(In4), Subsystem6/4(In4)
  Subsystem4/1(Out1) -> Out1/1
  Subsystem5/1(Out1) -> Out2/1
  Subsystem6/1(Out1) -> Out3/1
  Subsystem7/1(Out1) -> Out4/1

== system dandianji/control ==
  In1 : Inport
  Out1 : Outport
  wires:
  In1/1 -> Out1/1

== system dandianji/control1 ==
  Out1 : Outport

== system dandianji/control2 ==
  In1 : Inport
  In2 : Inport  Port=2
  In3 : Inport  Port=3
  In4 : Inport  Port=4
  Out1 : Outport
  wires:
  In1/1 -> Out1/1

== system dandianji/fuzzypid1 ==
  In1 : Inport
  Derivative : Derivative
  Subsystem : Subsystem
  Out1 : Outport
  wires:
  Subsystem/1(Out1) -> Out1/1
  Derivative/1 -> Subsystem/2(In2)
  In1/1 -> Derivative/1, Subsystem/1(In1)

== system dandianji/fuzzypid2 ==
  In1 : Inport
  Derivative : Derivative
  Subsystem : Subsystem
  Out1 : Outport
  wires:
  Subsystem/1(Out1) -> Out1/1
  Derivative/1 -> Subsystem/2(In2)
  In1/1 -> Derivative/1, Subsystem/1(In1)

== system dandianji/fuzzypid3 ==
  In1 : Inport
  Derivative : Derivative
  Subsystem : Subsystem
  Out1 : Outport
  wires:
  Subsystem/1(Out1) -> Out1/1
  Derivative/1 -> Subsystem/2(In2)
  In1/1 -> Derivative/1, Subsystem/1(In1)

== system dandianji/fuzzypid4 ==
  In1 : Inport
  Derivative : Derivative
  Subsystem : Subsystem
  Out1 : Outport
  wires:
  Subsystem/1(Out1) -> Out1/1
  Derivative/1 -> Subsystem/2(In2)
  In1/1 -> Derivative/1, Subsystem/1(In1)

== system dandianji/Subsystem4/Subsystem4 ==
  In1 : Inport
  In2 : Inport  Port=2
  In3 : Inport  Port=3
  In4 : Inport  Port=4
  Add : Sum  Inputs=+++
  PID Controller3 : simulink/Continuous/PID Controller  Controller=PID  TimeDomain=Continuous-time  SampleTime=-1  IntegratorMethod=Forward Euler  FilterMethod=Forward Euler  Form=Parallel  P=12.9851074749726  I=3.96505413373294  D=0.756963167778154  N=4061.73491108422  InitialConditionSource=internal  InitialConditionForIntegrator=0  InitialConditionForFilter=0  ExternalReset=none  LimitOutput=off  UpperSaturationLimit=inf  LowerSaturationLimit=-inf  LinearizeAsGain=on  AntiWindupMode=none  Kb=1  TrackingMode=off  Kt=1  PParamMin=[]  PParamMax=[]  IParamMin=[]  IParamMax=[]  DParamMin=[]  DParamMax=[]  NParamMin=[]  NParamMax=[]  KbParamMin=[]  KbParamMax=[]  KtParamMin=[]  KtParamMax=[]  POutMin=[]  POutMax=[]  IOutMin=[]  IOutMax=[]  DOutMin=[]  DOutMax=[]  NOutMin=[]  NOutMax=[]  KbOutMin=[]  KbOutMax=[]  KtOutMin=[]  KtOutMax=[]  IntegratorOutMin=[]  IntegratorOutMax=[]  FilterOutMin=[]  FilterOutMax=[]  SumOutMin=[]  SumOutMax=[]  SumI1OutMin=[]  SumI1OutMax=[]  SumI2OutMin=[]  SumI2OutMax=[]  SumI3OutMin=[]  SumI3OutMax=[]  SumDOutMin=[]  SumDOutMax=[]  SaturationOutMin=[]  SaturationOutMax=[]  IntegratorContinuousStateAttributes=''  IntegratorStateMustResolveToSignalObject=off  IntegratorRTWStateStorageClass=Auto  FilterContinuousStateAttributes=''  FilterStateMustResolveToSignalObject=off  FilterRTWStateStorageClass=Auto  DifferentiatorICPrevScaledInput=0  DifferentiatorOutMin=[]  DifferentiatorOutMax=[]  UseFilter=on
  PID Controller4 : simulink/Continuous/PID Controller  Controller=PID  TimeDomain=Continuous-time  SampleTime=-1  IntegratorMethod=Forward Euler  FilterMethod=Forward Euler  Form=Parallel  P=12.9851074749726  I=3.96505413373294  D=0.756963167778154  N=4061.73491108422  InitialConditionSource=internal  InitialConditionForIntegrator=0  InitialConditionForFilter=0  ExternalReset=none  LimitOutput=off  UpperSaturationLimit=inf  LowerSaturationLimit=-inf  LinearizeAsGain=on  AntiWindupMode=none  Kb=1  TrackingMode=off  Kt=1  PParamMin=[]  PParamMax=[]  IParamMin=[]  IParamMax=[]  DParamMin=[]  DParamMax=[]  NParamMin=[]  NParamMax=[]  KbParamMin=[]  KbParamMax=[]  KtParamMin=[]  KtParamMax=[]  POutMin=[]  POutMax=[]  IOutMin=[]  IOutMax=[]  DOutMin=[]  DOutMax=[]  NOutMin=[]  NOutMax=[]  KbOutMin=[]  KbOutMax=[]  KtOutMin=[]  KtOutMax=[]  IntegratorOutMin=[]  IntegratorOutMax=[]  FilterOutMin=[]  FilterOutMax=[]  SumOutMin=[]  SumOutMax=[]  SumI1OutMin=[]  SumI1OutMax=[]  SumI2OutMin=[]  SumI2OutMax=[]  SumI3OutMin=[]  SumI3OutMax=[]  SumDOutMin=[]  SumDOutMax=[]  SaturationOutMin=[]  SaturationOutMax=[]  IntegratorContinuousStateAttributes=''  IntegratorStateMustResolveToSignalObject=off  IntegratorRTWStateStorageClass=Auto  FilterContinuousStateAttributes=''  FilterStateMustResolveToSignalObject=off  FilterRTWStateStorageClass=Auto  DifferentiatorICPrevScaledInput=0  DifferentiatorOutMin=[]  DifferentiatorOutMax=[]  UseFilter=on
  PID Controller6 : simulink/Continuous/PID Controller  Controller=PID  TimeDomain=Continuous-time  SampleTime=-1  IntegratorMethod=Forward Euler  FilterMethod=Forward Euler  Form=Parallel  P=12.9851074749726  I=3.96505413373294  D=0.756963167778154  N=4061.73491108422  InitialConditionSource=internal  InitialConditionForIntegrator=0  InitialConditionForFilter=0  ExternalReset=none  LimitOutput=off  UpperSaturationLimit=inf  LowerSaturationLimit=-inf  LinearizeAsGain=on  AntiWindupMode=none  Kb=1  TrackingMode=off  Kt=1  PParamMin=[]  PParamMax=[]  IParamMin=[]  IParamMax=[]  DParamMin=[]  DParamMax=[]  NParamMin=[]  NParamMax=[]  KbParamMin=[]  KbParamMax=[]  KtParamMin=[]  KtParamMax=[]  POutMin=[]  POutMax=[]  IOutMin=[]  IOutMax=[]  DOutMin=[]  DOutMax=[]  NOutMin=[]  NOutMax=[]  KbOutMin=[]  KbOutMax=[]  KtOutMin=[]  KtOutMax=[]  IntegratorOutMin=[]  IntegratorOutMax=[]  FilterOutMin=[]  FilterOutMax=[]  SumOutMin=[]  SumOutMax=[]  SumI1OutMin=[]  SumI1OutMax=[]  SumI2OutMin=[]  SumI2OutMax=[]  SumI3OutMin=[]  SumI3OutMax=[]  SumDOutMin=[]  SumDOutMax=[]  SaturationOutMin=[]  SaturationOutMax=[]  IntegratorContinuousStateAttributes=''  IntegratorStateMustResolveToSignalObject=off  IntegratorRTWStateStorageClass=Auto  FilterContinuousStateAttributes=''  FilterStateMustResolveToSignalObject=off  FilterRTWStateStorageClass=Auto  DifferentiatorICPrevScaledInput=0  DifferentiatorOutMin=[]  DifferentiatorOutMax=[]  UseFilter=on
  Sum : Sum  Inputs=|+-
  Sum1 : Sum  Inputs=|+-
  Sum2 : Sum  Inputs=|+-
  fuzzypid1 : Subsystem
  fuzzypid2 : Subsystem
  fuzzypid3 : Subsystem
  Out1 : Outport
  wires:
  In1/1 -> Sum/1, Sum1/1, Sum2/1
  In2/1 -> Sum/2
  In3/1 -> Sum1/2
  In4/1 -> Sum2/2
  Sum/1 -> fuzzypid3/1(In1)
  Sum1/1 -> fuzzypid1/1(In1)
  Sum2/1 -> fuzzypid2/1(In1)
  Add/1 -> Out1/1
  fuzzypid3/1(Out1) -> Add/1
  fuzzypid1/1(Out1) -> Add/2
  fuzzypid2/1(Out1) -> Add/3

== system dandianji/Subsystem4/Subsystem5 ==
  In2 : Inport
  In1 : Inport  Port=2
  In3 : Inport  Port=3
  In4 : Inport  Port=4
  Add : Sum  Inputs=+++
  PID Controller1 : simulink/Continuous/PID Controller  Controller=PID  TimeDomain=Continuous-time  SampleTime=-1  IntegratorMethod=Forward Euler  FilterMethod=Forward Euler  Form=Parallel  P=12.9851074749726  I=3.96505413373294  D=0.756963167778154  N=4061.73491108422  InitialConditionSource=internal  InitialConditionForIntegrator=0  InitialConditionForFilter=0  ExternalReset=none  LimitOutput=off  UpperSaturationLimit=inf  LowerSaturationLimit=-inf  LinearizeAsGain=on  AntiWindupMode=none  Kb=1  TrackingMode=off  Kt=1  PParamMin=[]  PParamMax=[]  IParamMin=[]  IParamMax=[]  DParamMin=[]  DParamMax=[]  NParamMin=[]  NParamMax=[]  KbParamMin=[]  KbParamMax=[]  KtParamMin=[]  KtParamMax=[]  POutMin=[]  POutMax=[]  IOutMin=[]  IOutMax=[]  DOutMin=[]  DOutMax=[]  NOutMin=[]  NOutMax=[]  KbOutMin=[]  KbOutMax=[]  KtOutMin=[]  KtOutMax=[]  IntegratorOutMin=[]  IntegratorOutMax=[]  FilterOutMin=[]  FilterOutMax=[]  SumOutMin=[]  SumOutMax=[]  SumI1OutMin=[]  SumI1OutMax=[]  SumI2OutMin=[]  SumI2OutMax=[]  SumI3OutMin=[]  SumI3OutMax=[]  SumDOutMin=[]  SumDOutMax=[]  SaturationOutMin=[]  SaturationOutMax=[]  IntegratorContinuousStateAttributes=''  IntegratorStateMustResolveToSignalObject=off  IntegratorRTWStateStorageClass=Auto  FilterContinuousStateAttributes=''  FilterStateMustResolveToSignalObject=off  FilterRTWStateStorageClass=Auto  DifferentiatorICPrevScaledInput=0  DifferentiatorOutMin=[]  DifferentiatorOutMax=[]  UseFilter=on
  PID Controller2 : simulink/Continuous/PID Controller  Controller=PID  TimeDomain=Continuous-time  SampleTime=-1  IntegratorMethod=Forward Euler  FilterMethod=Forward Euler  Form=Parallel  P=12.9851074749726  I=3.96505413373294  D=0.756963167778154  N=4061.73491108422  InitialConditionSource=internal  InitialConditionForIntegrator=0  InitialConditionForFilter=0  ExternalReset=none  LimitOutput=off  UpperSaturationLimit=inf  LowerSaturationLimit=-inf  LinearizeAsGain=on  AntiWindupMode=none  Kb=1  TrackingMode=off  Kt=1  PParamMin=[]  PParamMax=[]  IParamMin=[]  IParamMax=[]  DParamMin=[]  DParamMax=[]  NParamMin=[]  NParamMax=[]  KbParamMin=[]  KbParamMax=[]  KtParamMin=[]  KtParamMax=[]  POutMin=[]  POutMax=[]  IOutMin=[]  IOutMax=[]  DOutMin=[]  DOutMax=[]  NOutMin=[]  NOutMax=[]  KbOutMin=[]  KbOutMax=[]  KtOutMin=[]  KtOutMax=[]  IntegratorOutMin=[]  IntegratorOutMax=[]  FilterOutMin=[]  FilterOutMax=[]  SumOutMin=[]  SumOutMax=[]  SumI1OutMin=[]  SumI1OutMax=[]  SumI2OutMin=[]  SumI2OutMax=[]  SumI3OutMin=[]  SumI3OutMax=[]  SumDOutMin=[]  SumDOutMax=[]  SaturationOutMin=[]  SaturationOutMax=[]  IntegratorContinuousStateAttributes=''  IntegratorStateMustResolveToSignalObject=off  IntegratorRTWStateStorageClass=Auto  FilterContinuousStateAttributes=''  FilterStateMustResolveToSignalObject=off  FilterRTWStateStorageClass=Auto  DifferentiatorICPrevScaledInput=0  DifferentiatorOutMin=[]  DifferentiatorOutMax=[]  UseFilter=on
  PID Controller5 : simulink/Continuous/PID Controller  Controller=PID  TimeDomain=Continuous-time  SampleTime=-1  IntegratorMethod=Forward Euler  FilterMethod=Forward Euler  Form=Parallel  P=12.9851074749726  I=3.96505413373294  D=0.756963167778154  N=4061.73491108422  InitialConditionSource=internal  InitialConditionForIntegrator=0  InitialConditionForFilter=0  ExternalReset=none  LimitOutput=off  UpperSaturationLimit=inf  LowerSaturationLimit=-inf  LinearizeAsGain=on  AntiWindupMode=none  Kb=1  TrackingMode=off  Kt=1  PParamMin=[]  PParamMax=[]  IParamMin=[]  IParamMax=[]  DParamMin=[]  DParamMax=[]  NParamMin=[]  NParamMax=[]  KbParamMin=[]  KbParamMax=[]  KtParamMin=[]  KtParamMax=[]  POutMin=[]  POutMax=[]  IOutMin=[]  IOutMax=[]  DOutMin=[]  DOutMax=[]  NOutMin=[]  NOutMax=[]  KbOutMin=[]  KbOutMax=[]  KtOutMin=[]  KtOutMax=[]  IntegratorOutMin=[]  IntegratorOutMax=[]  FilterOutMin=[]  FilterOutMax=[]  SumOutMin=[]  SumOutMax=[]  SumI1OutMin=[]  SumI1OutMax=[]  SumI2OutMin=[]  SumI2OutMax=[]  SumI3OutMin=[]  SumI3OutMax=[]  SumDOutMin=[]  SumDOutMax=[]  SaturationOutMin=[]  SaturationOutMax=[]  IntegratorContinuousStateAttributes=''  IntegratorStateMustResolveToSignalObject=off  IntegratorRTWStateStorageClass=Auto  FilterContinuousStateAttributes=''  FilterStateMustResolveToSignalObject=off  FilterRTWStateStorageClass=Auto  DifferentiatorICPrevScaledInput=0  DifferentiatorOutMin=[]  DifferentiatorOutMax=[]  UseFilter=on
  Sum : Sum  Inputs=|+-
  Sum1 : Sum  Inputs=|+-
  Sum2 : Sum  Inputs=|+-
  fuzzypid1 : Subsystem
  fuzzypid2 : Subsystem
  fuzzypid3 : Subsystem
  Out1 : Outport
  wires:
  In2/1 -> Sum/1, Sum1/1, Sum2/1
  In1/1 -> Sum/2
  In3/1 -> Sum1/2
  In4/1 -> Sum2/2
  Sum/1 -> fuzzypid3/1(In1)
  Sum1/1 -> fuzzypid1/1(In1)
  Sum2/1 -> fuzzypid2/1(In1)
  Add/1 -> Out1/1
  fuzzypid3/1(Out1) -> Add/1
  fuzzypid1/1(Out1) -> Add/2
  fuzzypid2/1(Out1) -> Add/3

== system dandianji/Subsystem4/Subsystem6 ==
  In3 : Inport
  In1 : Inport  Port=2
  In2 : Inport  Port=3
  In4 : Inport  Port=4
  Add : Sum  Inputs=+++
  PID Controller3 : simulink/Continuous/PID Controller  Controller=PID  TimeDomain=Continuous-time  SampleTime=-1  IntegratorMethod=Forward Euler  FilterMethod=Forward Euler  Form=Parallel  P=12.9851074749726  I=3.96505413373294  D=0.756963167778154  N=4061.73491108422  InitialConditionSource=internal  InitialConditionForIntegrator=0  InitialConditionForFilter=0  ExternalReset=none  LimitOutput=off  UpperSaturationLimit=inf  LowerSaturationLimit=-inf  LinearizeAsGain=on  AntiWindupMode=none  Kb=1  TrackingMode=off  Kt=1  PParamMin=[]  PParamMax=[]  IParamMin=[]  IParamMax=[]  DParamMin=[]  DParamMax=[]  NParamMin=[]  NParamMax=[]  KbParamMin=[]  KbParamMax=[]  KtParamMin=[]  KtParamMax=[]  POutMin=[]  POutMax=[]  IOutMin=[]  IOutMax=[]  DOutMin=[]  DOutMax=[]  NOutMin=[]  NOutMax=[]  KbOutMin=[]  KbOutMax=[]  KtOutMin=[]  KtOutMax=[]  IntegratorOutMin=[]  IntegratorOutMax=[]  FilterOutMin=[]  FilterOutMax=[]  SumOutMin=[]  SumOutMax=[]  SumI1OutMin=[]  SumI1OutMax=[]  SumI2OutMin=[]  SumI2OutMax=[]  SumI3OutMin=[]  SumI3OutMax=[]  SumDOutMin=[]  SumDOutMax=[]  SaturationOutMin=[]  SaturationOutMax=[]  IntegratorContinuousStateAttributes=''  IntegratorStateMustResolveToSignalObject=off  IntegratorRTWStateStorageClass=Auto  FilterContinuousStateAttributes=''  FilterStateMustResolveToSignalObject=off  FilterRTWStateStorageClass=Auto  DifferentiatorICPrevScaledInput=0  DifferentiatorOutMin=[]  DifferentiatorOutMax=[]  UseFilter=on
  PID Controller4 : simulink/Continuous/PID Controller  Controller=PID  TimeDomain=Continuous-time  SampleTime=-1  IntegratorMethod=Forward Euler  FilterMethod=Forward Euler  Form=Parallel  P=12.9851074749726  I=3.96505413373294  D=0.756963167778154  N=4061.73491108422  InitialConditionSource=internal  InitialConditionForIntegrator=0  InitialConditionForFilter=0  ExternalReset=none  LimitOutput=off  UpperSaturationLimit=inf  LowerSaturationLimit=-inf  LinearizeAsGain=on  AntiWindupMode=none  Kb=1  TrackingMode=off  Kt=1  PParamMin=[]  PParamMax=[]  IParamMin=[]  IParamMax=[]  DParamMin=[]  DParamMax=[]  NParamMin=[]  NParamMax=[]  KbParamMin=[]  KbParamMax=[]  KtParamMin=[]  KtParamMax=[]  POutMin=[]  POutMax=[]  IOutMin=[]  IOutMax=[]  DOutMin=[]  DOutMax=[]  NOutMin=[]  NOutMax=[]  KbOutMin=[]  KbOutMax=[]  KtOutMin=[]  KtOutMax=[]  IntegratorOutMin=[]  IntegratorOutMax=[]  FilterOutMin=[]  FilterOutMax=[]  SumOutMin=[]  SumOutMax=[]  SumI1OutMin=[]  SumI1OutMax=[]  SumI2OutMin=[]  SumI2OutMax=[]  SumI3OutMin=[]  SumI3OutMax=[]  SumDOutMin=[]  SumDOutMax=[]  SaturationOutMin=[]  SaturationOutMax=[]  IntegratorContinuousStateAttributes=''  IntegratorStateMustResolveToSignalObject=off  IntegratorRTWStateStorageClass=Auto  FilterContinuousStateAttributes=''  FilterStateMustResolveToSignalObject=off  FilterRTWStateStorageClass=Auto  DifferentiatorICPrevScaledInput=0  DifferentiatorOutMin=[]  DifferentiatorOutMax=[]  UseFilter=on
  PID Controller6 : simulink/Continuous/PID Controller  Controller=PID  TimeDomain=Continuous-time  SampleTime=-1  IntegratorMethod=Forward Euler  FilterMethod=Forward Euler  Form=Parallel  P=12.9851074749726  I=3.96505413373294  D=0.756963167778154  N=4061.73491108422  InitialConditionSource=internal  InitialConditionForIntegrator=0  InitialConditionForFilter=0  ExternalReset=none  LimitOutput=off  UpperSaturationLimit=inf  LowerSaturationLimit=-inf  LinearizeAsGain=on  AntiWindupMode=none  Kb=1  TrackingMode=off  Kt=1  PParamMin=[]  PParamMax=[]  IParamMin=[]  IParamMax=[]  DParamMin=[]  DParamMax=[]  NParamMin=[]  NParamMax=[]  KbParamMin=[]  KbParamMax=[]  KtParamMin=[]  KtParamMax=[]  POutMin=[]  POutMax=[]  IOutMin=[]  IOutMax=[]  DOutMin=[]  DOutMax=[]  NOutMin=[]  NOutMax=[]  KbOutMin=[]  KbOutMax=[]  KtOutMin=[]  KtOutMax=[]  IntegratorOutMin=[]  IntegratorOutMax=[]  FilterOutMin=[]  FilterOutMax=[]  SumOutMin=[]  SumOutMax=[]  SumI1OutMin=[]  SumI1OutMax=[]  SumI2OutMin=[]  SumI2OutMax=[]  SumI3OutMin=[]  SumI3OutMax=[]  SumDOutMin=[]  SumDOutMax=[]  SaturationOutMin=[]  SaturationOutMax=[]  IntegratorContinuousStateAttributes=''  IntegratorStateMustResolveToSignalObject=off  IntegratorRTWStateStorageClass=Auto  FilterContinuousStateAttributes=''  FilterStateMustResolveToSignalObject=off  FilterRTWStateStorageClass=Auto  DifferentiatorICPrevScaledInput=0  DifferentiatorOutMin=[]  DifferentiatorOutMax=[]  UseFilter=on
  Sum : Sum  Inputs=|+-
  Sum1 : Sum  Inputs=|+-
  Sum2 : Sum  Inputs=|+-
  fuzzypid1 : Subsystem
  fuzzypid2 : Subsystem
  fuzzypid3 : Subsystem
  Out1 : Outport
  wires:
  In3/1 -> Sum/1, Sum1/1, Sum2/1
  In1/1 -> Sum/2
  In2/1 -> Sum1/2
  In4/1 -> Sum2/2
  Sum/1 -> fuzzypid3/1(In1)
  Sum1/1 -> fuzzypid1/1(In1)
  Sum2/1 -> fuzzypid2/1(In1)
  Add/1 -> Out1/1
  fuzzypid3/1(Out1) -> Add/1
  fuzzypid1/1(Out1) -> Add/2
  fuzzypid2/1(Out1) -> Add/3
